simulink model "FloatShield_LQ"  (R2019a)
settings: Solver=FixedStepDiscrete  StartTime=0.0  StopTime=Inf  FixedStep=0.025  RelTol=1e-3  EnableMultiTasking=on
undefined symbols (not defined in the file): Discrete, RefVect, Time
libraries: simulink x1, arduinolib x1, ctrlSharedLib x1, dspmathops x1
settings Model: SimulationMode=external  ExtModeTrigDuration=2  Creator=Peter  LastModifiedBy=Gergely
settings OptimizationCC: EnhancedBackFolding=on  PassReuseOutputArgsAs=Individual arguments  MaxStackSize=64  OptimizeBlockOrder=speed  DifferentSizesBufferReuse=on  OptimizationCustomize=off
settings DebuggingCC: ParameterTunabilityLossMsg=error
settings HardwareCC: ProdBitPerInt=16  ProdBitPerPointer=16  ProdBitPerSizeT=16  ProdBitPerPtrDiffT=16  ProdLargestAtomicFloat=None  ProdWordSize=8  ProdHWDeviceType=Atmel->AVR
settings SFSimCC: MATLABDynamicMemAlloc=off
settings RTWCC: SystemTargetFile=ert.tlc  HardwareBoard=Arduino Uno  TLCOptions=-aInlineSetEventsForThisBaseRateFcn=TLC_FALSE -aSuppressMultiTaskScheduler=TLC_FALSE -aRateBasedStepFcn=1  TemplateMakefile=ert_default_tmf  GenerateReport=on  Toolchain=Arduino AVR  BuildConfiguration=Faster Runs  IncludeHyperlinkInReport=on  LaunchReport=on  GenerateTraceInfo=on  GenerateTraceReport=on  GenerateTraceReportSl=on  GenerateTraceReportSf=on  GenerateTraceReportEml=on
settings CodeAppCC: ForceParamTrailComments=on  IgnoreCustomStorageClasses=off  OperatorAnnotations=on  SimulinkDataObjDesc=on  SFDataObjDesc=on  InsertBlockDesc=on
settings ERTTargetCC: SupportContinuousTime=on  SupportVariableSizeSignals=on  ExtModeStaticAllocSize=250

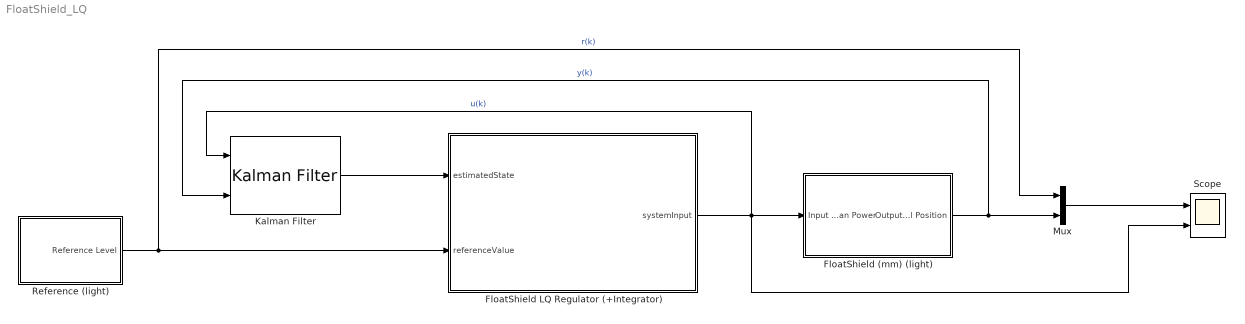
== system FloatShield_LQ ==
  FloatShield (mm) (light) : Subsystem  mask{CalTime=5, Ts=0.025}
      mask prompts: CalTime "Calibration time (s):"; Ts "Sampling period (s):"
      mask DialogControl DescGroupVar Prompt: FloatShield
      mask DialogControl DescTextVar Prompt: The block represents the FloatShield device. It accepts an input signal in the range of 0-100% that controls the fan power level and outputs ball position as an altitude in millimetres. The block performs calibration at the start of simulation for a defined period of time. This is more memory-friendly version of the block.
      mask DialogControl defVal Prompt: Default values
      mask DialogControl defVal Callback:
      | CurrentBlock = gcb;
      | set_param(CurrentBlock,'CalTime','5');
      | set_param(CurrentBlock,'Ts','0.025');
      mask Display: image('assets\FloatShield.svg');
  FloatShield LQ Regulator (+Integrator) : Subsystem  mask{gainK=[0.4582, 0.1997, 0.6398, -0.0025], Ts=0.025}
      mask prompts: gainK "LQ gain matrix K:"; Ts "Sampling period (s):"
      mask DialogControl DescGroupVar Prompt: LQ regulator
      mask DialogControl DescTextVar Prompt: Block representing LQ regulator reaslised using MATLAB Function block. Regulator includes integrator as its fourth state. Can be used only with three state systems (plus integrator as fourth), as it was created purely for FloatShield application.
      mask DialogControl defVal Prompt: Default values
      mask DialogControl defVal Callback:
      | CurrentBlock = gcb;
      | set_param(CurrentBlock,'gainK','[0.4582, 0.1997, 0.6398, -0.0025]');
      | set_param(CurrentBlock,'Ts','0.025');
  Kalman Filter : ctrlSharedLib/Kalman Filter  TimeDomain=Discrete-Time  UseCurrentEstimator=on  ModelSource=Individual A, B, C, D matrices  ModelSourceVariable=ss(0.95,1,1,0,1)  A=[1, 0.0244, 0.0006; 0, 0.9502, 0.0472; 0, 0, 0.8987]  B=[0.0001; 0.0132; 0.5168]  C=[1, 0, 0]  D=0  NumberOfStates=1  NumberOfInputs=1  NumberOfOutputs=1  InitialEstimateSource=Dialog  X0=[0;0;0]  P0=10  UseK=off  UseGH=off  NumberOfProcessNoiseInputs=1  G=1  TimeInvariantG=on  H=0  TimeInvariantH=on  Q=[5, 0, 0; 0, 1000, 0; 0, 0, 1000]  TimeInvariantQ=on  R=25  TimeInvariantR=on  N=0  TimeInvariantN=on  AddInputPort=on  AddEnablePort=off  OutputEstimatedY=off  OutputP=off  Ts=-1
  Mux : Mux  Inputs=2
  Reference (light) : Subsystem  StopFcn=|  mask{RefVect=[210,160,110,145,195,245,180,130,65,95], RefLen=length(RefVect), SectLen=30, Ts=0.025}
      | if exist('ScopeData')
      | structVar=ScopeData;
      | end
      | 
      | if exist('structVar')
      | [a u]=structVar.signals.values;
      | r=a(:,1);
      | y=a(:,2);
      | SimulinkLQResponse=[r,y,u];
      | clear ScopeData structVar a u r y ;
      | save SimulinkLQResponse SimulinkLQResponse;
      | plotResults(SimulinkLQResponse);
      | end
      mask prompts: RefVect "Reference vector:"; RefLen "Reference vector length"; SectLen "Section duration (s):"; Ts "Sampling period (s):"
      mask init:
      | RefLen = length(RefVect);
      mask DialogControl DescGroupVar Prompt: Reference Block (light)
      mask DialogControl DescTextVar Prompt: Block used to provide changing reference levels during simulation. This is more memory-friendly version of the block.
      mask DialogControl defVal Prompt: Default values
      mask DialogControl defVal Callback:
      | CurrentBlock = gcb;
      | set_param(CurrentBlock,'RefVect','[210,160,110,145,195,245,180,130,65,95]');
      | set_param(CurrentBlock,'SectLen','30');
      | set_param(CurrentBlock,'Ts','0.025');
  Scope : Scope  NumInputPorts=2
  wires:
  Mux/1 -> Scope/1
  FloatShield LQ Regulator (+Integrator)/1(systemInput) -> Scope/2, Kalman Filter/1, FloatShield (mm) (light)/1(Input Fan Power)  "u(k)"
  Reference (light)/1(Reference Level) -> FloatShield LQ Regulator (+Integrator)/2(referenceValue), Mux/1  "r(k)"
  FloatShield (mm) (light)/1(Output Ball Position) -> Kalman Filter/2, Mux/2  "y(k)"
  Kalman Filter/1 -> FloatShield LQ Regulator (+Integrator)/1(estimatedState)

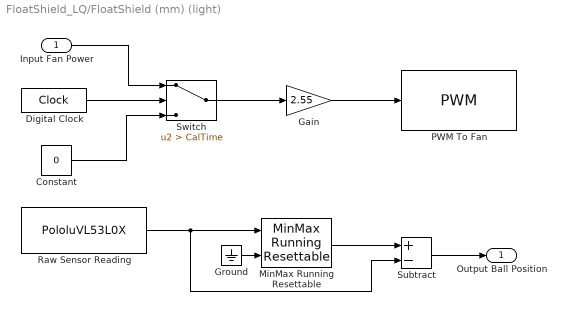
== system FloatShield_LQ/FloatShield (mm) (light) ==
  Input Fan Power : Inport  SampleTime=Ts
  Constant : Constant  Value=0  SampleTime=Ts
  Digital Clock : DigitalClock  SampleTime=Ts
  Gain : Gain  Gain=2.55
  Ground : Ground
  MinMax Running Resettable : simulink/Math Operations/MinMax Running Resettable  Function=max  vinit=150
  PWM To Fan : arduinolib/PWM  pinNumber=3  frequencyType=Default  desiredFrequency=490.2  achievableFrequency=490.2
  Raw Sensor Reading : S-Function  FunctionName=PololuVL53L0X  SFunctionModules='PololuVL53L0X_wrapper'  SFunctionDeploymentMode=off  EnableBusSupport=off
  Subtract : Sum  Inputs=+-
  Switch : Switch  Criteria=u2 > Threshold  Threshold=CalTime
  Output Ball Position : Outport  SampleTime=Ts  VectorParamsAs1DForOutWhenUnconnected=off
  wires:
  Ground/1 -> MinMax Running Resettable/2
  MinMax Running Resettable/1 -> Subtract/1
  Raw Sensor Reading/1 -> MinMax Running Resettable/1, Subtract/2
  Constant/1 -> Switch/3
  Gain/1 -> PWM To Fan/1
  Switch/1 -> Gain/1
  Digital Clock/1 -> Switch/2
  Subtract/1 -> Output Ball Position/1
  Input Fan Power/1 -> Switch/1

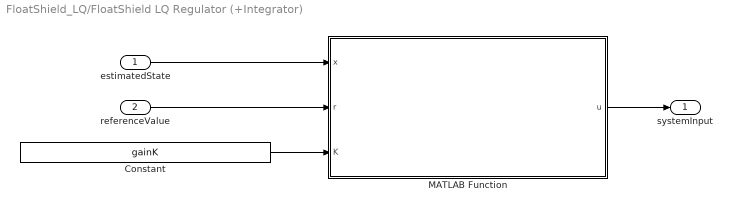
== system FloatShield_LQ/FloatShield LQ Regulator (+Integrator) ==
  estimatedState : Inport  SampleTime=Ts
  referenceValue : Inport  Port=2  SampleTime=Ts
  Constant : Constant  Value=gainK  VectorParams1D=off  SampleTime=Ts
  MATLAB Function : MATLAB Function  TreatAsAtomicUnit=on
  systemInput : Outport  SampleTime=Ts  VectorParamsAs1DForOutWhenUnconnected=off
  wires:
  Constant/1 -> MATLAB Function/3(K)
  referenceValue/1 -> MATLAB Function/2(r)
  MATLAB Function/1(u) -> systemInput/1
  estimatedState/1 -> MATLAB Function/1(x)

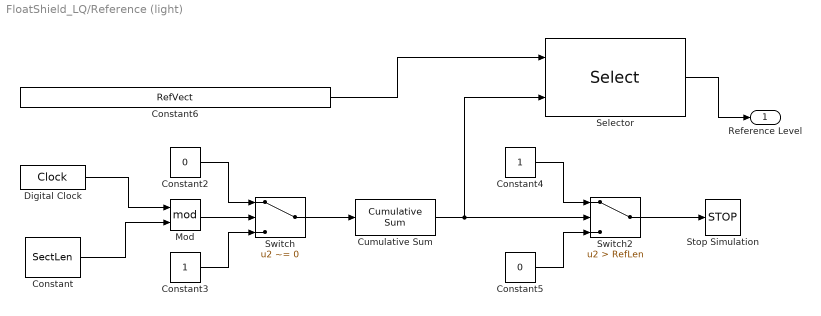
== system FloatShield_LQ/Reference (light) ==
  Constant : Constant  Value=SectLen  SampleTime=Ts
  Constant2 : Constant  Value=0  SampleTime=Ts
  Constant3 : Constant  SampleTime=Ts
  Constant4 : Constant  SampleTime=Ts
  Constant5 : Constant  Value=0  SampleTime=Ts
  Constant6 : Constant  Value=RefVect  SampleTime=Ts
  Cumulative Sum : dspmathops/Cumulative Sum  dim=Channels (running sum)  InputProcessing=Columns as channels (frame based)  reset_popup=None  roundingMode=Floor  overflowMode=off  outputDataTypeStr=Inherit: Same as accumulator  outputMin=[]  outputMax=[]  outputLastDataTypeStr=Inherit: Same as accumulator
  Digital Clock : DigitalClock  SampleTime=Ts
  Mod : Math  Operator=mod  SaturateOnIntegerOverflow=on
  Selector : Selector  InputPortWidth=RefLen  IndexOptions=Index vector (port)  Indices=[1 3]  OutputSizes=1
  Stop Simulation : Stop
  Switch : Switch  Criteria=u2 ~= 0
  Switch2 : Switch  Criteria=u2 > Threshold  Threshold=RefLen  OutDataTypeStr=Inherit: Inherit via back propagation
  Reference Level : Outport  SampleTime=Ts  VectorParamsAs1DForOutWhenUnconnected=off
  wires:
  Constant4/1 -> Switch2/1
  Mod/1 -> Switch/2
  Digital Clock/1 -> Mod/1
  Cumulative Sum/1 -> Switch2/2, Selector/2
  Selector/1 -> Reference Level/1
  Constant6/1 -> Selector/1
  Constant/1 -> Mod/2
  Constant5/1 -> Switch2/3
  Constant2/1 -> Switch/1
  Switch2/1 -> Stop Simulation/1
  Switch/1 -> Cumulative Sum/1
  Constant3/1 -> Switch/3

== matlab function FloatShield_LQ/FloatShield LQ Regulator (+Integrator)/MATLAB Function ==
  data: x input; u output; r input; K input
function u = fcn(x, r, K)
persistent xI;
if isempty(xI)    
    xI = 0;
end
xI = xI + r - x(1);
x = [x; xI];
u = -K * (x - [r;0;0;0]);
